simulink model "Spacecraft_Attitude_Dynamics_Control"  (R2020a)
settings: Solver=FixedStepDiscrete  StartTime=0.0  StopTime=300  FixedStep=dt  MaxStep=dt  RelTol=1e-3  EnableMultiTasking=on
InitFcn:
  | % No [0 0 1] %polar orbit
  | 
  | clc
  | close all
  | clear all
  | r0 = [6678;0;0]; %km
  | mu = 398600.4418; % km^3/sec^2
  | v0 = sqrt(mu/norm(r0))*[0;1;0]; % km/s
  | T0 = [0; 0; 0];
  | 
  | I1 = 3;
  | I2 = 4;
  | I3 = 2;
  | I = [I1 0 0; 0 I2 0; 0 0 I3];
  | Iinv  = I ^-1;
  | 
  | k1 = (I1 - I3)/I2;
  | k2 = (I2 - I3)/I1;
  | k3 = (I2 - I1)/I3;
  | n = sqrt(mu/norm(r0)^3);
  | 
  | A11 = zeros(3,3);
  | A12 = (1/2)*eye(3);
  | 
  | F = [-8*k1*n^2 0 0; 0 -6*k2*n^2 0; 0 0 -2*k3*n^2];
  | G = [0 0 (1-k1)*n; 0 0 0; (k3 - 1)*n 0 0];
  | 
  | A = [A11 A12; F G];
  | 
  | B1 = zeros(3,3);
  | B2 =[1/I1 0 0; 0 1/I2 0; 0 0 1/I3];
  | 
  | B = [B1; B2];
  | 
  | Q = [0.32 0 0 0 0 0;
  |        0 0.36 0 0 0 0;
  |        0 0 0.3 0 0 0;
  |        0 0 0 180 0 0;
  |        0 0 0 0 190 0;
  |        0 0 0 0 0 11.5]*10^-4;
  | 
  | 
  | R_LQR = eye(3);
  | 
  | Rinv = R_LQR\eye(3);
  | 
  | S = care(A,B,Q,R_LQR);
  | 
  | K = Rinv*B'*S;
  | 
  | dt = 0.005;
  | dtsim = 0.1;
  | dtdata = 0.01;
  | dtcontrol = 0.2;
  | 
  | Tdist = 0*ones(3,1);
  | Tmin = -0.001; %Nm
  | Tmax = 0.001; %Nm
  | 
  | qTarget = [1;0;0;0];
  | 
  | w0 = [0;0;0]; % Tip: Set w0 to no motion.
  | 
  | H0 = [0;0;0];
  | R = -pi/4;
  | P = pi/4;
  | Y = pi/3;
  | 
  | m = [-0.05; -0.03; -0.05];
  | d = [10; 10 ;10]*(pi/180);
  | 
  | q0 = [cos(R/2)*cos(P/2)*cos(Y/2) - sin(R/2)*sin(P/2)*sin(Y/2);
  |          sin(R/2)*cos(P/2)*cos(Y/2) + cos(R/2)*sin(P/2)*sin(Y/2);
  |          cos(R/2)*sin(P/2)*cos(Y/2) - sin(R/2)*cos(P/2)*sin(Y/2);
  |          cos(R/2)*cos(P/2)*sin(Y/2) + sin(R/2)*sin(P/2)*cos(Y/2)];
  | 
  | 
  | myworld = vrworld('SpacecraftEarth.wrl');
  | open(myworld);
  | set(0,'Units','pixels');
  | scnsize = get(0,'ScreenSize');
  | f1 = vrfigure(myworld,[1 80 scnsize(3)/2 scnsize(4)/2]);
  | set(f1,'Viewpoint','WorldView')
  | f2 = vrfigure(myworld,[scnsize(3)/2 80 scnsize(3)/2 scnsize(4)/2]);
  | set(f2,'Viewpoint','BodyView')
StopFcn:
  | % Roll vs. Time
  | figure
  | 
  | subplot(3,3,1)
  | plot(RPY.time, RPY.signals.values(:,1), '-k');
  | hold on
  | plot([0 RPY.time(end)], 5 *pi/180 * [1,1],'-r');
  | plot([0 RPY.time(end)], -5 *pi/180 * [1,1],'-r');
  | xlabel('Time, sec')
  | ylabel('Roll, rad')
  | xlim([0 RPY.time(end)])
  | hold off
  | 
  | subplot(3,3,2)
  | plot(RPY.time, RPY.signals.values(:,2), '-k');
  | hold on
  | plot([0 RPY.time(end)], 5 *pi/180 * [1,1],'-r');
  | plot([0 RPY.time(end)], -5 *pi/180 * [1,1],'-r');
  | xlabel('Time, sec')
  | ylabel('Pitch, rad')
  | xlim([0 RPY.time(end)])
  | hold off
  | 
  | subplot(3,3,3)
  | plot(RPY.time, RPY.signals.values(:,3), '-k');
  | hold on
  | plot([0 RPY.time(end)], 5 *pi/180 * [1,1],'-r');
  | plot([0 RPY.time(end)], -5 *pi/180 * [1,1],'-r');
  | xlabel('Time, sec')
  | ylabel('Yaw, rad')
  | xlim([0 RPY.time(end)])
  | hold off
  | 
  | % Roll Torque vs. Time
  | subplot(3,3,4)
  | hold on;
  | plot(Torque.time, Torque.signals.values(:,1), '-k');
  | xlabel('Time (seconds)');
  | ylabel('Roll Torque (Newton-Meters)');
  | xlim([0 Torque.time(end)]);
  | 
  | % Pitch Torque vs. Time
  | subplot(3,3,5)
  | hold on;
  | plot(Torque.time, Torque.signals.values(:,2), '-k');
  | xlabel('Time (seconds)');
  | ylabel('Pitch Torque (Newton-Meters)');
  | xlim([0 Torque.time(end)]);
  | 
  | % Yaw Torque vs. Time
  | subplot(3,3,6)
  | hold on;
  | plot(Torque.time, Torque.signals.values(:,3), '-k');
  | xlabel('Time (seconds)');
  | ylabel('Yaw Torque (Newton-Meters)');
  | xlim([0 Torque.time(end)]);
  | 
  | subplot(3,3,7)
  | hold on;
  | plot(thetaError.signals.values(:,1),thetaDot.signals.values(:,1),'-k');
  | axis manual;
  | pause(0.1);
  | plot([-2 2], [m(1)*-2+m(1)*d(1)/2, m(1)*2+m(1)*d(1)/2],'-r');
  | plot([-2 2], [m(1)*-2-m(1)*d(1)/2, m(1)*2-m(1)*d(1)/2],'-r');
  | 
  | 
  | subplot(3,3,8)
  | hold on;
  | plot(thetaError.signals.values(:,2),thetaDot.signals.values(:,2),'-k');
  | axis manual;
  | pause(0.1);
  | plot([-2 2], [m(2)*-2+m(2)*d(2)/2, m(2)*2+m(2)*d(2)/2],'-r');
  | plot([-2 2], [m(2)*-2-m(2)*d(2)/2, m(2)*2-m(2)*d(2)/2],'-r');
  | 
  | 
  | subplot(3,3,9)
  | hold on;
  | plot(thetaError.signals.values(:,3),thetaDot.signals.values(:,3),'-k');
  | axis manual;
  | pause(0.1);
  | plot([-2 2], [m(3)*-2+m(3)*d(3)/2, m(3)*2+m(3)*d(3)/2],'-r');
  | plot([-2 2], [m(3)*-2-m(3)*d(3)/2, m(3)*2-m(3)*d(3)/2],'-r');
  | hold off
  | 
  | 
  | titletext = ['Cost Function J = ' num2str(J.signals.values(end))];
  | sgtitle(titletext)
  | fprintf('%d %d %d \n',abs(RPY.signals.values(end,:)*180/pi)<0.1)
  | fprintf('%d %d %d \n',abs(thetaDot.signals.values(end,1:3))<1e-4)
  | display(RPY.signals.values(end,:)*180/pi)
  | display(thetaDot.signals.values(end,1:3))
undefined symbols (not defined in the file): DiscIntNeverNeededParam
libraries: sharedutil x5, vrlib x1, simulink x1
settings Model: Creator=HANE  LastModifiedBy=Edward Han
settings DataIOCC: ReturnWorkspaceOutputs=off
settings DebuggingCC: SFExecutionAtInitializationDiag=none  ArithmeticOperatorsInVariantConditions=warning
settings SFSimCC: SimUseLocalCustomCode=off  CustomCodeUndefinedFunction=UseInterfaceOnly
settings RTWCC: RTWUseLocalCustomCode=off
settings CodeAppCC: StateflowObjectComments=on

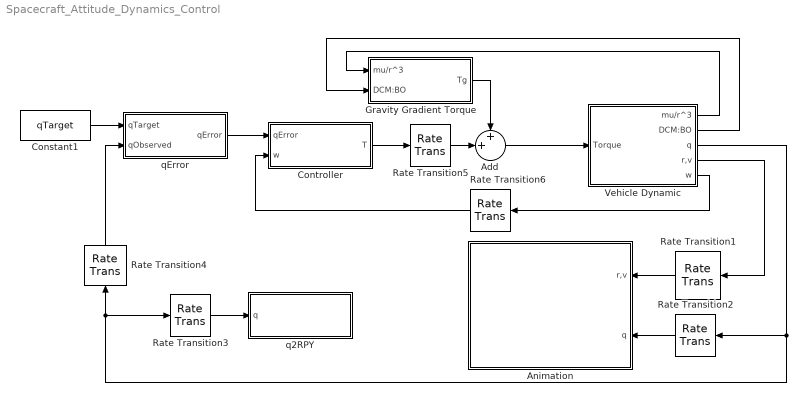
== system Spacecraft_Attitude_Dynamics_Control ==
  Add : Sum  Inputs=++|
  Animation : Subsystem
  Constant1 : Constant  Value=qTarget
  Controller : Subsystem
  Gravity Gradient Torque : Subsystem
  Rate Transition1 : RateTransition  InitialCondition=[r0;v0]  OutPortSampleTime=dtsim
  Rate Transition2 : RateTransition  InitialCondition=q0  OutPortSampleTime=dtsim
  Rate Transition3 : RateTransition  InitialCondition=q0  OutPortSampleTime=dtdata
  Rate Transition4 : RateTransition  InitialCondition=q0  OutPortSampleTime=dtcontrol
  Rate Transition5 : RateTransition  InitialCondition=T0  OutPortSampleTime=dt
  Rate Transition6 : RateTransition  InitialCondition=w0  OutPortSampleTime=dtcontrol
  Vehicle Dynamic : Subsystem
  q2RPY : Subsystem
  qError : Subsystem
  wires:
  Add/1 -> Vehicle Dynamic/1(Torque)
  Vehicle Dynamic/4(r,v) -> Rate Transition1/1
  Vehicle Dynamic/3(q) -> Rate Transition3/1, Rate Transition4/1, Rate Transition2/1
  Rate Transition2/1 -> Animation/2(q)
  Rate Transition1/1 -> Animation/1(r,v)
  Rate Transition3/1 -> q2RPY/1(q)
  Rate Transition5/1 -> Add/2
  Controller/1(T) -> Rate Transition5/1
  Constant1/1 -> qError/1(qTarget)
  qError/1(qError) -> Controller/1(qError)
  Rate Transition4/1 -> qError/2(qObserved)
  Vehicle Dynamic/5(w) -> Rate Transition6/1
  Vehicle Dynamic/1(mu/r^3) -> Gravity Gradient Torque/1(mu/r^3)
  Vehicle Dynamic/2(DCM:BO) -> Gravity Gradient Torque/2(DCM:BO)
  Gravity Gradient Torque/1(Tg) -> Add/1
  Rate Transition6/1 -> Controller/2("w ")

== system Spacecraft_Attitude_Dynamics_Control/Animation ==
  r,v : Inport
  q : Inport  Port=2
  Demux : Demux  Outputs=[3,3]
  Earth Rotation : Subsystem
  VR Sink : vrlib/VR Sink  InstantiateOnLoad=on  SampleTime=dtsim  ViewEnable=on  RemoteChange=off  RemoteView=off  FieldsWritten=Earth.rotation.4.1.1.double#BodyView.orientation.4.1.1.double#BodyView.position.3.1.1.double#Spacecraft.rotation.4.1.1.double#Spacecraft.translation.3.1.1.double  WorldFileName=SpacecraftEarth.wrl  AutoView=off  VideoDimensions=[]  AllowVariableSize=off
  q2eulerparameters : Subsystem
  qBody wrt Inertial : Subsystem
  qOrbit wrt Inertial : Subsystem
  qOrbit wrt Inertial1 : Subsystem
  "r, translation" : Subsystem
  wires:
  Demux/1 -> qOrbit wrt Inertial/1(r), "r, translation"/1(r), qOrbit wrt Inertial1/1(r)
  Demux/2 -> qOrbit wrt Inertial/2(v)
  q/1 -> qBody wrt Inertial/2(qBO)
  qOrbit wrt Inertial/2("qOI ") -> qBody wrt Inertial/1(qOI)
  qBody wrt Inertial/1(qBI) -> q2eulerparameters/1(q)
  r,v/1 -> Demux/1
  "r, translation"/1(translation) -> VR Sink/5
  qOrbit wrt Inertial/1(DCM) -> qOrbit wrt Inertial1/2(DCM)
  Earth Rotation/1(Earth Rotation) -> VR Sink/1
  qOrbit wrt Inertial1/1(Nadir View Rotation) -> VR Sink/2
  qOrbit wrt Inertial1/2(Nadir View Position) -> VR Sink/3
  q2eulerparameters/1(e,phi) -> VR Sink/4

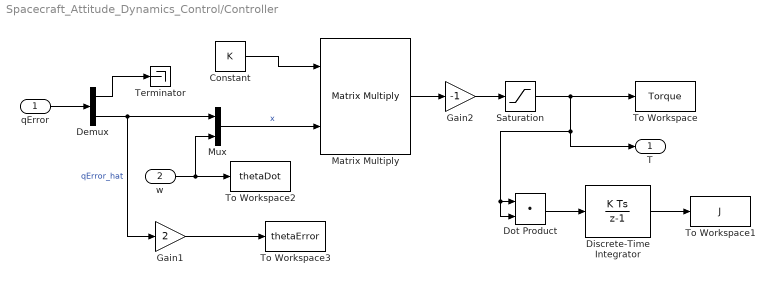
== system Spacecraft_Attitude_Dynamics_Control/Controller ==
  qError : Inport  SampleTime=dtcontrol
  "w " : Inport  Port=2
  Constant : Constant  Value=K
  Demux : Demux  Outputs=[1,3]
  Discrete-Time Integrator : DiscreteIntegrator  SampleTime=dtcontrol  ICPrevOutput=DiscIntNeverNeededParam  ICPrevScaledInput=DiscIntNeverNeededParam
  Dot Product : DotProduct  InputSameDT=on  OutDataTypeStr=Inherit: Inherit via internal rule
  Gain1 : Gain  Gain=2
  Gain2 : Gain  Gain=-1
  Matrix Multiply : Product  Multiplication=Matrix(*)
  Mux : Mux  Inputs=2
  Saturation : Saturate  UpperLimit=Tmax  LowerLimit=-Tmax
  Terminator : Terminator
  To Workspace : ToWorkspace  VariableName=Torque  SaveFormat=Structure With Time  SampleTime=-1
  To Workspace1 : ToWorkspace  VariableName=J  SaveFormat=Structure With Time  SampleTime=-1
  To Workspace2 : ToWorkspace  VariableName=thetaDot  SaveFormat=Structure With Time  SampleTime=-1
  To Workspace3 : ToWorkspace  VariableName=thetaError  SaveFormat=Structure With Time  SampleTime=-1
  T : Outport  VectorParamsAs1DForOutWhenUnconnected=off
  wires:
  qError/1 -> Demux/1
  "w "/1 -> To Workspace2/1, Mux/2
  Demux/2 -> Gain1/1, Mux/1  "qError_hat"
  Demux/1 -> Terminator/1
  Mux/1 -> Matrix Multiply/2  "x"
  Matrix Multiply/1 -> Gain2/1
  Gain2/1 -> Saturation/1
  Dot Product/1 -> Discrete-Time Integrator/1
  Discrete-Time Integrator/1 -> To Workspace1/1
  Constant/1 -> Matrix Multiply/1
  Gain1/1 -> To Workspace3/1
  Saturation/1 -> To Workspace/1, Dot Product/2, Dot Product/1, T/1

== system Spacecraft_Attitude_Dynamics_Control/Gravity Gradient Torque ==
  mu/r^3 : Inport
  DCM:BO : Inport  Port=2
  3x3 Cross Product : sharedutil/3x3 Cross Product  aMode=aMode
      settings: SourceProductBaseCode=AE,PW,MT,VE,VP
  Constant : Constant  Value=[0;0;-1]
  Gain : Gain  Gain=3
  "I " : Constant  Value=I
  Matrix Multiply : Product  Multiplication=Matrix(*)
  Multiply : Product
  Multiply1 : Product  Multiplication=Matrix(*)
  Tg : Outport  VectorParamsAs1DForOutWhenUnconnected=off
  wires:
  mu/r^3/1 -> Gain/1
  DCM:BO/1 -> Matrix Multiply/1
  Constant/1 -> Matrix Multiply/2
  Matrix Multiply/1 -> Multiply1/2, Multiply/2  "rhat"
  Gain/1 -> Multiply/1
  Multiply/1 -> 3x3 Cross Product/1
  3x3 Cross Product/1 -> Tg/1
  "I "/1 -> Multiply1/1
  Multiply1/1 -> 3x3 Cross Product/2

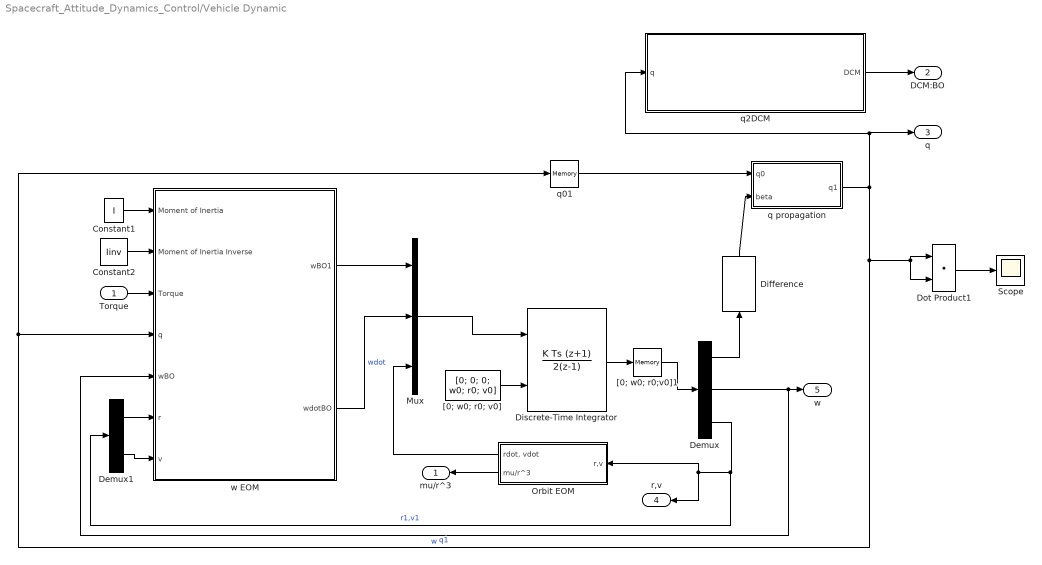
== system Spacecraft_Attitude_Dynamics_Control/Vehicle Dynamic ==
  Torque : Inport
  Constant1 : Constant  Value=I
  Constant2 : Constant  Value=Iinv
  Demux : Demux  Outputs=[3,3,6]
  Demux1 : Demux  Outputs=2
  Difference : simulink/Discrete/Difference  ICPrevInput=0.0  OutMin=[]  OutMax=[]  OutDataType=fixdt(1, 16)  OutScaling=2^-10  DoSatur=off
  Discrete-Time Integrator : DiscreteIntegrator  IntegratorMethod=Integration: Trapezoidal  InitialConditionSource=external  SampleTime=dt  ICPrevOutput=DiscIntNeverNeededParam  ICPrevScaledInput=DiscIntNeverNeededParam
  Dot Product1 : DotProduct  InputSameDT=on  OutDataTypeStr=Inherit: Inherit via internal rule
  Mux : Mux  Inputs=3
  Orbit EOM : Subsystem
  Scope : Scope
  "[0; w0; r0; v0]" : Constant  Value=[0; 0; 0; w0; r0; v0]
  "[0; w0; r0;v0]1" : Memory  InitialCondition=[0; 0; 0; w0; r0; v0]  InheritSampleTime=on
  q propagation : Subsystem
  q01 : Memory  InitialCondition=q0  InheritSampleTime=on
  q2DCM : Subsystem
  w EOM : Subsystem
  mu/r^3 : Outport  VectorParamsAs1DForOutWhenUnconnected=off
  DCM:BO : Outport  Port=2  VectorParamsAs1DForOutWhenUnconnected=off
  q : Outport  Port=3  VectorParamsAs1DForOutWhenUnconnected=off
  r,v : Outport  Port=4  VectorParamsAs1DForOutWhenUnconnected=off
  w : Outport  Port=5  VectorParamsAs1DForOutWhenUnconnected=off
  wires:
  Mux/1 -> Discrete-Time Integrator/1
  Demux/3 -> Demux1/1, Orbit EOM/1(r,v), r,v/1  "r1,v1"
  Constant1/1 -> w EOM/1(Moment of Inertia)
  "[0; w0; r0;v0]1"/1 -> Demux/1
  "[0; w0; r0; v0]"/1 -> Discrete-Time Integrator/2
  Orbit EOM/1("rdot, vdot ") -> Mux/3
  Torque/1 -> w EOM/3(Torque)
  q propagation/1(q1) -> Dot Product1/1, Dot Product1/2, q01/1, w EOM/4(q), q/1, q2DCM/1(q)  "q1"
  Difference/1 -> q propagation/2(beta)
  q01/1 -> q propagation/1(q0)
  Constant2/1 -> w EOM/2(Moment of Inertia Inverse)
  Dot Product1/1 -> Scope/1
  Discrete-Time Integrator/1 -> "[0; w0; r0;v0]1"/1
  w EOM/2(wdotBO) -> Mux/2  "wdot"
  Demux1/2 -> w EOM/7("v ")
  Demux1/1 -> w EOM/6(r)
  Demux/2 -> w/1, w EOM/5("wBO ")  "w"
  Demux/1 -> Difference/1
  w EOM/1(wBO1) -> Mux/1
  q2DCM/1(DCM) -> DCM:BO/1
  Orbit EOM/2(mu/r^3) -> mu/r^3/1

== system Spacecraft_Attitude_Dynamics_Control/q2RPY ==
  q : Inport
  DCM(1,1) : Fcn  Expr=(u(1)^2+u(2)^2-u(3)^2-u(4)^2)
  DCM(2,1) : Fcn  Expr=2*(u(2)*u(3)-u(4)*u(1))
  DCM(3,1) : Fcn  Expr=2*(u(2)*u(4)+u(1)*u(3))
  DCM(3,2) : Fcn  Expr=2*(u(3)*u(4)-u(1)*u(2))
  DCM(3,3) : Fcn  Expr=(u(1)^2-u(2)^2-u(3)^2+u(4)^2)
  Gain : Gain  Gain=-1
  Gain1 : Gain  Gain=-1
  Mux : Mux  Inputs=3
  To Workspace : ToWorkspace  VariableName=RPY  SaveFormat=Structure With Time  SampleTime=-1
  Trigonometric Function : Trigonometry  Operator=asin
  Trigonometric Function1 : Trigonometry  Operator=atan2
  Trigonometric Function2 : Trigonometry  Operator=atan2
  wires:
  q/1 -> DCM(1,1)/1, DCM(2,1)/1, DCM(3,3)/1, DCM(3,2)/1, DCM(3,1)/1
  DCM(3,1)/1 -> Trigonometric Function/1
  DCM(3,3)/1 -> Trigonometric Function1/2
  Trigonometric Function1/1 -> Mux/1  "R"
  Trigonometric Function/1 -> Mux/2  "P"
  DCM(1,1)/1 -> Trigonometric Function2/2
  Trigonometric Function2/1 -> Mux/3  "Y"
  Mux/1 -> To Workspace/1
  Gain/1 -> Trigonometric Function2/1
  DCM(2,1)/1 -> Gain/1
  DCM(3,2)/1 -> Gain1/1
  Gain1/1 -> Trigonometric Function1/1

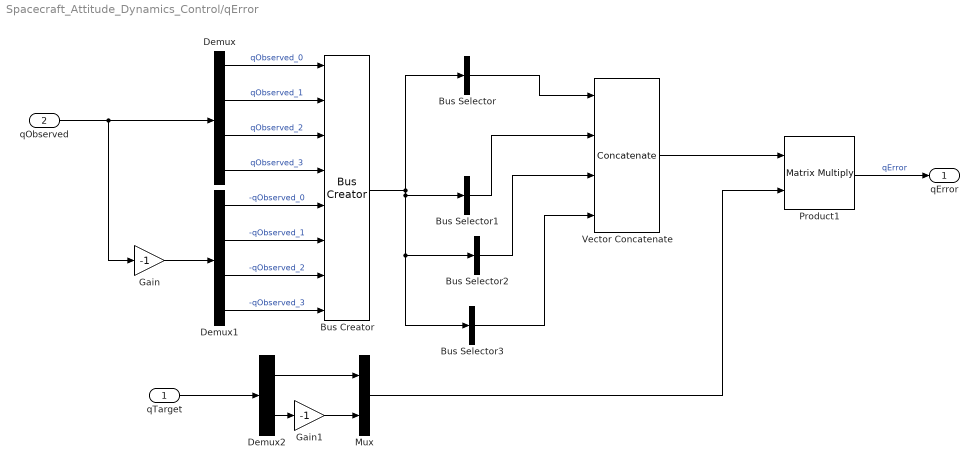
== system Spacecraft_Attitude_Dynamics_Control/qError ==
  qTarget : Inport
  qObserved : Inport  Port=2
  Bus Creator : BusCreator  Inputs=8
  Bus Selector : BusSelector  OutputSignals=qObserved_0,qObserved_1,qObserved_2,qObserved_3  OutputAsBus=on
  Bus Selector1 : BusSelector  OutputSignals=-qObserved_1,qObserved_0,-qObserved_3,qObserved_2  OutputAsBus=on
  Bus Selector2 : BusSelector  OutputSignals=-qObserved_2,qObserved_3,qObserved_0,-qObserved_1  OutputAsBus=on
  Bus Selector3 : BusSelector  OutputSignals=-qObserved_3,-qObserved_2,qObserved_1,qObserved_0  OutputAsBus=on
  Demux : Demux
  Demux1 : Demux
  Demux2 : Demux  Outputs=[1,3]
  Gain : Gain  Gain=-1
  Gain1 : Gain  Gain=-1
  Mux : Mux  Inputs=2
  Product1 : Product  Multiplication=Matrix(*)
  Vector Concatenate : Concatenate  NumInputs=4  Mode=Multidimensional array  ConcatenateDimension=2
  qError : Outport  VectorParamsAs1DForOutWhenUnconnected=off
  wires:
  qObserved/1 -> Gain/1, Demux/1
  Bus Selector3/1 -> Vector Concatenate/4
  Bus Selector2/1 -> Vector Concatenate/3
  Bus Creator/1 -> Bus Selector/1, Bus Selector2/1, Bus Selector3/1, Bus Selector1/1
  Demux1/2 -> Bus Creator/6  "-qObserved_1"
  Mux/1 -> Product1/2
  Product1/1 -> qError/1  "qError"
  Vector Concatenate/1 -> Product1/1
  Demux/2 -> Bus Creator/2  "qObserved_1"
  Bus Selector1/1 -> Vector Concatenate/2
  Demux1/1 -> Bus Creator/5  "-qObserved_0"
  Demux1/4 -> Bus Creator/8  "-qObserved_3"
  Demux/4 -> Bus Creator/4  "qObserved_3"
  Demux/3 -> Bus Creator/3  "qObserved_2"
  Gain/1 -> Demux1/1
  Bus Selector/1 -> Vector Concatenate/1
  Demux/1 -> Bus Creator/1  "qObserved_0"
  Demux1/3 -> Bus Creator/7  "-qObserved_2"
  qTarget/1 -> Demux2/1
  Demux2/2 -> Gain1/1
  Demux2/1 -> Mux/1
  Gain1/1 -> Mux/2

== system Spacecraft_Attitude_Dynamics_Control/Animation/Earth Rotation ==
  Cos : Trigonometry  Operator=cos
  Digital Clock : DigitalClock  SampleTime=dtsim
  Gain : Gain  Gain=1/2
  Gain1 : Gain  Gain=1/sqrt(2)
  Mux : Mux
  Product : Product
  Sin : Trigonometry
  q2eulerparameters : Subsystem
  w Earth : Constant  Value=2*pi/(24*3600)
  Earth Rotation : Outport  VectorParamsAs1DForOutWhenUnconnected=off
  wires:
  Gain1/1 -> q2eulerparameters/1(q)
  Cos/1 -> Mux/2, Mux/1
  Sin/1 -> Mux/4, Mux/3
  Mux/1 -> Gain1/1
  q2eulerparameters/1(e,phi) -> Earth Rotation/1
  Gain/1 -> Sin/1, Cos/1
  Product/1 -> Gain/1
  w Earth/1 -> Product/2
  Digital Clock/1 -> Product/1

== system Spacecraft_Attitude_Dynamics_Control/Animation/q2eulerparameters ==
  q : Inport
  Demux : Demux  Outputs=[1,3]
  Divide : Product  Inputs=/*
  Gain : Gain  Gain=2
  Mux : Mux  Inputs=2
  Trigonometric Function : Trigonometry  Operator=acos
  Trigonometric Function1 : Trigonometry
  e,phi : Outport  VectorParamsAs1DForOutWhenUnconnected=off
  wires:
  Demux/2 -> Divide/2  "qhat"
  Trigonometric Function1/1 -> Divide/1
  Divide/1 -> Mux/1  "e"
  Trigonometric Function/1 -> Trigonometric Function1/1, Gain/1  "phi/2"
  Demux/1 -> Trigonometric Function/1  "q0"
  Gain/1 -> Mux/2  "phi"
  Mux/1 -> e,phi/1
  q/1 -> Demux/1

== system Spacecraft_Attitude_Dynamics_Control/Animation/qBody wrt Inertial ==
  qOI : Inport
  qBO : Inport  Port=2
  Bus Creator : BusCreator  Inputs=8
  Bus Selector : BusSelector  OutputSignals=qBO_0,qBO_1,qBO_2,qBO_3  OutputAsBus=on
  Bus Selector1 : BusSelector  OutputSignals=-qBO_1,qBO_0,-qBO_3,qBO_2  OutputAsBus=on
  Bus Selector2 : BusSelector  OutputSignals=-qBO_2,qBO_3,qBO_0,-qBO_1  OutputAsBus=on
  Bus Selector3 : BusSelector  OutputSignals=-qBO_3,-qBO_2,qBO_1,qBO_0  OutputAsBus=on
  Demux : Demux
  Demux1 : Demux
  Gain : Gain  Gain=-1
  Product1 : Product  Multiplication=Matrix(*)
  Vector Concatenate : Concatenate  NumInputs=4  Mode=Multidimensional array  ConcatenateDimension=2
  qBI : Outport  VectorParamsAs1DForOutWhenUnconnected=off
  wires:
  qBO/1 -> Demux/1, Gain/1
  Demux/1 -> Bus Creator/1  "qBO_0"
  Gain/1 -> Demux1/1
  Demux/2 -> Bus Creator/2  "qBO_1"
  Demux/3 -> Bus Creator/3  "qBO_2"
  Demux/4 -> Bus Creator/4  "qBO_3"
  Demux1/1 -> Bus Creator/5  "-qBO_0"
  Demux1/2 -> Bus Creator/6  "-qBO_1"
  Demux1/3 -> Bus Creator/7  "-qBO_2"
  Demux1/4 -> Bus Creator/8  "-qBO_3"
  Bus Creator/1 -> Bus Selector3/1, Bus Selector2/1, Bus Selector1/1, Bus Selector/1
  Bus Selector3/1 -> Vector Concatenate/4
  Bus Selector2/1 -> Vector Concatenate/3
  Bus Selector1/1 -> Vector Concatenate/2
  Bus Selector/1 -> Vector Concatenate/1
  Vector Concatenate/1 -> Product1/1
  qOI/1 -> Product1/2
  Product1/1 -> qBI/1  "qBI"

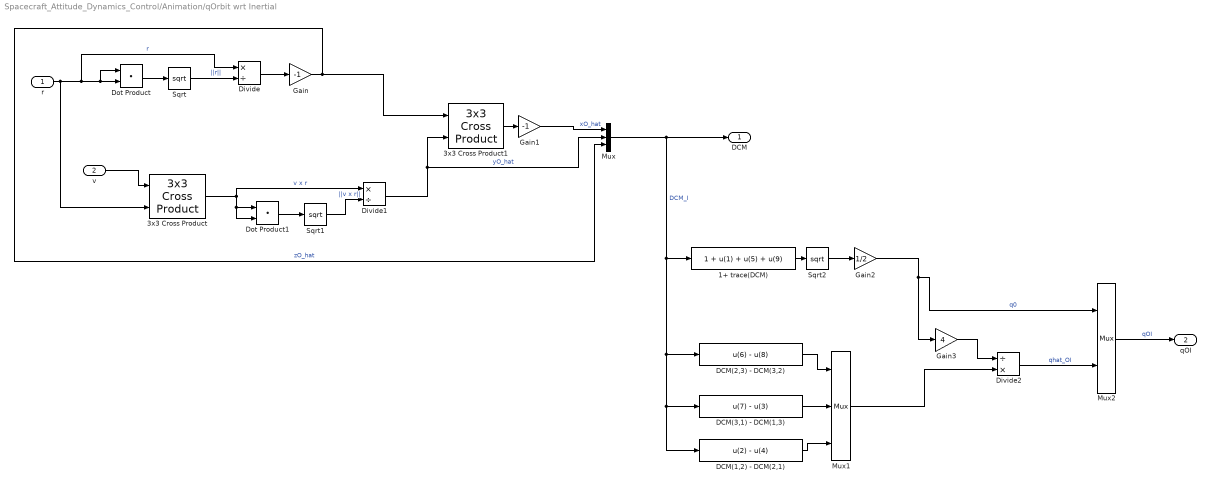
== system Spacecraft_Attitude_Dynamics_Control/Animation/qOrbit wrt Inertial ==
  r : Inport
  v : Inport  Port=2
  "1+ trace(DCM) " : Fcn  Expr=1 + u(1) + u(5) + u(9)
  3x3 Cross Product : sharedutil/3x3 Cross Product  aMode=aMode
      settings: SourceProductBaseCode=AE,PW,MT,VE,VP
  3x3 Cross Product1 : sharedutil/3x3 Cross Product  aMode=aMode
      settings: SourceProductBaseCode=AE,PW,MT,VE,VP
  DCM(1,2) - DCM(2,1) : Fcn  Expr=u(2) - u(4)
  DCM(2,3) - DCM(3,2) : Fcn  Expr=u(6) - u(8)
  DCM(3,1) - DCM(1,3) : Fcn  Expr=u(7) - u(3)
  Divide : Product  Inputs=*/
  Divide1 : Product  Inputs=*/
  Divide2 : Product  Inputs=/*
  Dot Product : DotProduct  InputSameDT=on  OutDataTypeStr=Inherit: Inherit via internal rule
  Dot Product1 : DotProduct  InputSameDT=on  OutDataTypeStr=Inherit: Inherit via internal rule
  Gain : Gain  Gain=-1
  Gain1 : Gain  Gain=-1
  Gain2 : Gain  Gain=1/2
  Gain3 : Gain  Gain=4
  Mux : Mux  Inputs=3
  Mux1 : Mux  Inputs=3
  Mux2 : Mux  Inputs=2
  Sqrt : Sqrt  SaturateOnIntegerOverflow=on
  Sqrt1 : Sqrt  SaturateOnIntegerOverflow=on
  Sqrt2 : Sqrt  SaturateOnIntegerOverflow=on
  DCM : Outport  VectorParamsAs1DForOutWhenUnconnected=off
  "qOI " : Outport  Port=2  VectorParamsAs1DForOutWhenUnconnected=off
  wires:
  Sqrt/1 -> Divide/2  "||r||"
  r/1 -> 3x3 Cross Product/2, Divide/1, Dot Product/1, Dot Product/2  "r"
  Dot Product/1 -> Sqrt/1
  Divide/1 -> Gain/1
  Gain/1 -> 3x3 Cross Product1/1, Mux/3  "zO_hat"
  v/1 -> 3x3 Cross Product/1
  Dot Product1/1 -> Sqrt1/1
  Sqrt1/1 -> Divide1/2  "||v x r||"
  3x3 Cross Product/1 -> Dot Product1/1, Dot Product1/2, Divide1/1  "v x r"
  Divide1/1 -> 3x3 Cross Product1/2, Mux/2  "yO_hat"
  3x3 Cross Product1/1 -> Gain1/1
  Gain1/1 -> Mux/1  "xO_hat"
  Mux/1 -> DCM(3,1) - DCM(1,3)/1, DCM(1,2) - DCM(2,1)/1, DCM(2,3) - DCM(3,2)/1, "1+ trace(DCM) "/1, DCM/1  "DCM_I"
  "1+ trace(DCM) "/1 -> Sqrt2/1
  Sqrt2/1 -> Gain2/1
  Gain2/1 -> Mux2/1, Gain3/1  "q0"
  DCM(2,3) - DCM(3,2)/1 -> Mux1/1
  DCM(3,1) - DCM(1,3)/1 -> Mux1/2
  DCM(1,2) - DCM(2,1)/1 -> Mux1/3
  Gain3/1 -> Divide2/1
  Mux1/1 -> Divide2/2
  Divide2/1 -> Mux2/2  "qhat_OI"
  Mux2/1 -> "qOI "/1  "qOI"

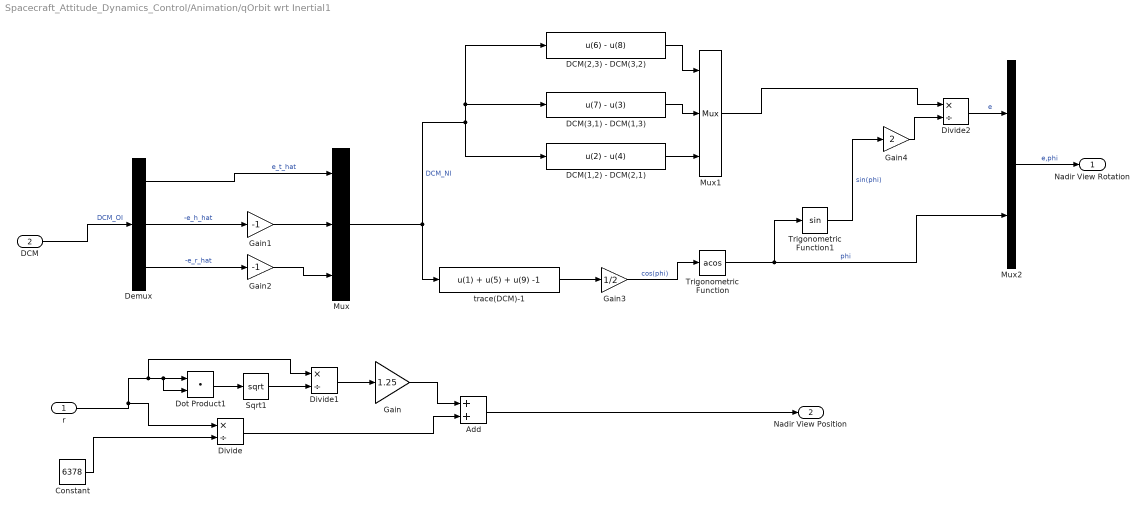
== system Spacecraft_Attitude_Dynamics_Control/Animation/qOrbit wrt Inertial1 ==
  r : Inport
  DCM : Inport  Port=2
  Add : Sum
  Constant : Constant  Value=6378
  DCM(1,2) - DCM(2,1) : Fcn  Expr=u(2) - u(4)
  DCM(2,3) - DCM(3,2) : Fcn  Expr=u(6) - u(8)
  DCM(3,1) - DCM(1,3) : Fcn  Expr=u(7) - u(3)
  Demux : Demux  Outputs=[3,3,3]
  Divide : Product  Inputs=*/
  Divide1 : Product  Inputs=*/
  Divide2 : Product  Inputs=*/
  Dot Product1 : DotProduct  InputSameDT=on  OutDataTypeStr=Inherit: Inherit via internal rule
  Gain : Gain  Gain=1.25
  Gain1 : Gain  Gain=-1
  Gain2 : Gain  Gain=-1
  Gain3 : Gain  Gain=1/2
  Gain4 : Gain  Gain=2
  Mux : Mux  Inputs=3
  Mux1 : Mux  Inputs=3
  Mux2 : Mux  Inputs=2
  Sqrt1 : Sqrt  SaturateOnIntegerOverflow=on
  Trigonometric Function : Trigonometry  Operator=acos
  Trigonometric Function1 : Trigonometry
  "trace(DCM)-1 " : Fcn  Expr=u(1) + u(5) + u(9) -1
  Nadir View Rotation : Outport  VectorParamsAs1DForOutWhenUnconnected=off
  Nadir View Position : Outport  Port=2  VectorParamsAs1DForOutWhenUnconnected=off
  wires:
  Constant/1 -> Divide/2
  Add/1 -> Nadir View Position/1
  r/1 -> Divide1/1, Dot Product1/2, Dot Product1/1, Divide/1
  Divide/1 -> Add/2
  Sqrt1/1 -> Divide1/2
  Dot Product1/1 -> Sqrt1/1
  Divide1/1 -> Gain/1
  Gain/1 -> Add/1
  DCM/1 -> Demux/1  "DCM_OI"
  Demux/1 -> Mux/1  "e_t_hat"
  Demux/2 -> Gain1/1  "-e_h_hat"
  Demux/3 -> Gain2/1  "-e_r_hat"
  Gain1/1 -> Mux/2
  Gain2/1 -> Mux/3
  Mux/1 -> DCM(3,1) - DCM(1,3)/1, DCM(2,3) - DCM(3,2)/1, DCM(1,2) - DCM(2,1)/1, "trace(DCM)-1 "/1  "DCM_NI"
  DCM(3,1) - DCM(1,3)/1 -> Mux1/2
  "trace(DCM)-1 "/1 -> Gain3/1
  DCM(1,2) - DCM(2,1)/1 -> Mux1/3
  Divide2/1 -> Mux2/1  "e"
  DCM(2,3) - DCM(3,2)/1 -> Mux1/1
  Gain3/1 -> Trigonometric Function/1  "cos(phi)"
  Trigonometric Function/1 -> Mux2/2, Trigonometric Function1/1  "phi"
  Trigonometric Function1/1 -> Gain4/1  "sin(phi)"
  Gain4/1 -> Divide2/2
  Mux1/1 -> Divide2/1
  Mux2/1 -> Nadir View Rotation/1  "e,phi"

== system Spacecraft_Attitude_Dynamics_Control/Animation/r, translation ==
  r : Inport
  Constant : Constant  Value=6378
  Divide : Product  Inputs=*/
  translation : Outport  VectorParamsAs1DForOutWhenUnconnected=off
  wires:
  r/1 -> Divide/1
  Divide/1 -> translation/1
  Constant/1 -> Divide/2

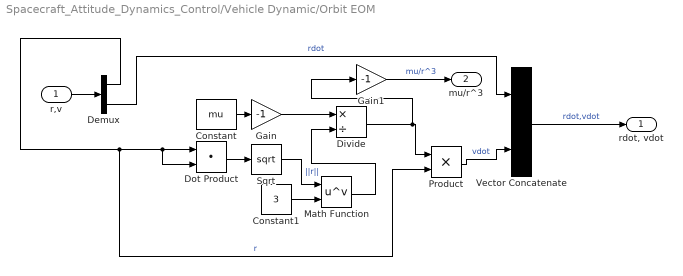
== system Spacecraft_Attitude_Dynamics_Control/Vehicle Dynamic/Orbit EOM ==
  r,v : Inport
  Constant : Constant  Value=mu
  Constant1 : Constant  Value=3
  Demux : Demux  Outputs=[3,3]
  Divide : Product  Inputs=*/
  Dot Product : DotProduct  InputSameDT=on  OutDataTypeStr=Inherit: Inherit via internal rule
  Gain : Gain  Gain=-1
  Gain1 : Gain  Gain=-1
  Math Function : Math  Operator=pow  SignedPower=on  SaturateOnIntegerOverflow=on
  Product : Product
  Sqrt : Sqrt  SaturateOnIntegerOverflow=on
  Vector Concatenate : Concatenate
  "rdot, vdot " : Outport  VectorParamsAs1DForOutWhenUnconnected=off
  mu/r^3 : Outport  Port=2  VectorParamsAs1DForOutWhenUnconnected=off
  wires:
  Dot Product/1 -> Sqrt/1
  Sqrt/1 -> Math Function/1  "||r||"
  Constant1/1 -> Math Function/2
  Math Function/1 -> Divide/2
  Constant/1 -> Gain/1
  Gain/1 -> Divide/1
  Divide/1 -> Gain1/1, Product/1
  Product/1 -> Vector Concatenate/2  "vdot"
  Vector Concatenate/1 -> "rdot, vdot "/1  "rdot,vdot"
  r,v/1 -> Demux/1
  Demux/1 -> Product/2, Dot Product/2, Dot Product/1  "r"
  Demux/2 -> Vector Concatenate/1  "rdot"
  Gain1/1 -> mu/r^3/1  "mu/r^3"

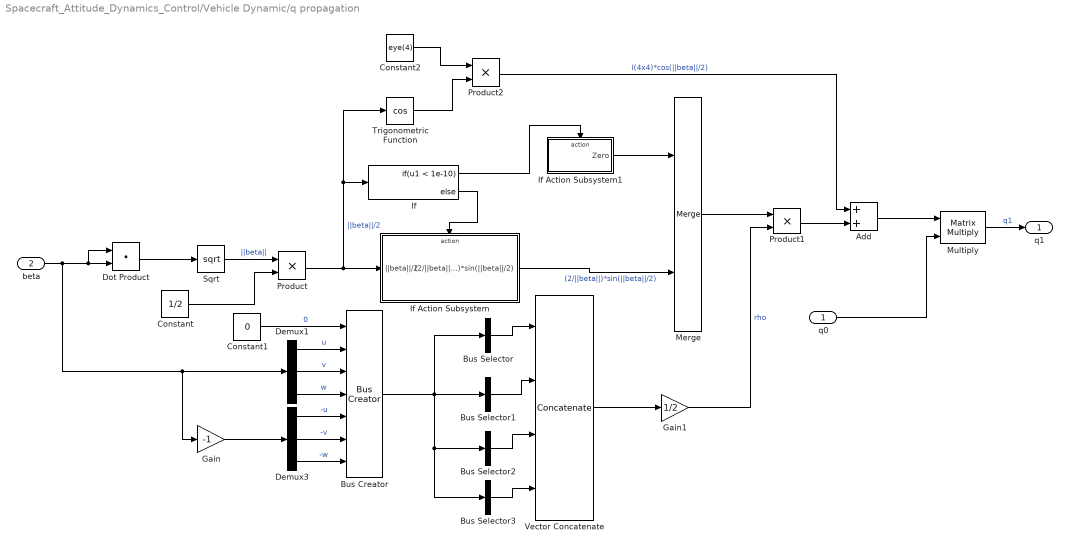
== system Spacecraft_Attitude_Dynamics_Control/Vehicle Dynamic/q propagation ==
  q0 : Inport
  beta : Inport  Port=2
  Add : Sum
  Bus Creator : BusCreator  Inputs=7
  Bus Selector : BusSelector  OutputSignals=0,u,v,w  OutputAsBus=on
  Bus Selector1 : BusSelector  OutputSignals=-u,0,-w,v  OutputAsBus=on
  Bus Selector2 : BusSelector  OutputSignals=-v,w,0,-u  OutputAsBus=on
  Bus Selector3 : BusSelector  OutputSignals=-w,-v,u,0  OutputAsBus=on
  Constant : Constant  Value=1/2
  Constant1 : Constant  Value=0
  Constant2 : Constant  Value=eye(4)
  Demux1 : Demux  Outputs=3
      settings: DisplayOption=none
  Demux3 : Demux  Outputs=3
      settings: DisplayOption=none
  Dot Product : DotProduct  InputSameDT=on  OutDataTypeStr=Inherit: Inherit via internal rule
  Gain : Gain  Gain=-1
  Gain1 : Gain  Gain=1/2
  If : If  IfExpression=u1 < 1e-10
  If Action Subsystem : Subsystem  TreatAsAtomicUnit=on
  If Action Subsystem1 : Subsystem  TreatAsAtomicUnit=on
  Merge : Merge
  Multiply : Product  Multiplication=Matrix(*)
  Product : Product
  Product1 : Product
  Product2 : Product
  Sqrt : Sqrt  SaturateOnIntegerOverflow=on
  Trigonometric Function : Trigonometry  Operator=cos
  Vector Concatenate : Concatenate  NumInputs=4  Mode=Multidimensional array  ConcatenateDimension=2
  q1 : Outport  VectorParamsAs1DForOutWhenUnconnected=off
  wires:
  If/1 -> If Action Subsystem1/Action
  If/2 -> If Action Subsystem/Action
  Merge/1 -> Product1/1
  If Action Subsystem1/1(Zero) -> Merge/1
  Product/1 -> Trigonometric Function/1, If/1, If Action Subsystem/1(||beta||/2)  "||beta||/2"
  If Action Subsystem/1((2/||beta||)*sin(||beta||/2)) -> Merge/2  "(2/||beta||)*sin(||beta||/2)"
  Sqrt/1 -> Product/1  "||beta||"
  beta/1 -> Gain/1, Demux1/1, Dot Product/1, Dot Product/2
  Dot Product/1 -> Sqrt/1
  Constant/1 -> Product/2
  Gain/1 -> Demux3/1
  Demux1/2 -> Bus Creator/3  "v"
  Demux1/1 -> Bus Creator/2  "u"
  Demux1/3 -> Bus Creator/4  "w"
  Demux3/1 -> Bus Creator/5  "-u"
  Demux3/2 -> Bus Creator/6  "-v"
  Demux3/3 -> Bus Creator/7  "-w"
  Constant1/1 -> Bus Creator/1  "0"
  Bus Creator/1 -> Bus Selector3/1, Bus Selector2/1, Bus Selector1/1, Bus Selector/1
  Bus Selector/1 -> Vector Concatenate/1
  Bus Selector1/1 -> Vector Concatenate/2
  Bus Selector2/1 -> Vector Concatenate/3
  Bus Selector3/1 -> Vector Concatenate/4
  Vector Concatenate/1 -> Gain1/1
  Gain1/1 -> Product1/2  "rho"
  Constant2/1 -> Product2/1
  Trigonometric Function/1 -> Product2/2
  Product2/1 -> Add/1  "I(4x4)*cos(||beta||/2)"
  Product1/1 -> Add/2
  Add/1 -> Multiply/1
  q0/1 -> Multiply/2
  Multiply/1 -> q1/1  "q1"

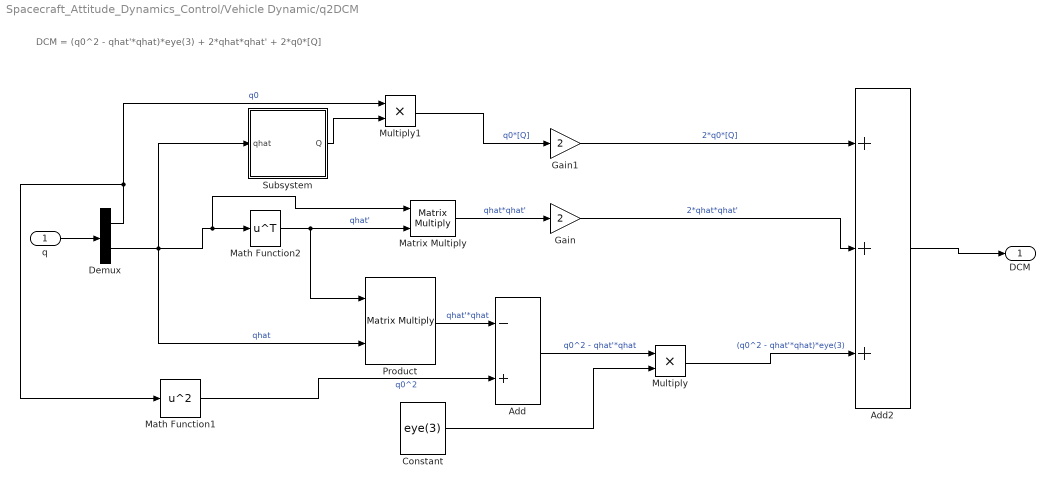
== system Spacecraft_Attitude_Dynamics_Control/Vehicle Dynamic/q2DCM ==
  note: DCM = (q0^2 - qhat'*qhat)*eye(3) + 2*qhat*qhat' + 2*q0*[Q]
  q : Inport  PortDimensions=[4,1]
  Add : Sum  Inputs=-+
  Add2 : Sum  Inputs=+++
  Constant : Constant  Value=eye(3)
  Demux : Demux  Outputs=[1,3]
  Gain : Gain  Gain=2
  Gain1 : Gain  Gain=2
  Math Function1 : Math  Operator=square  SignedPower=on  SaturateOnIntegerOverflow=on
  Math Function2 : Math  Operator=transpose  SignedPower=on  SaturateOnIntegerOverflow=on
  Matrix Multiply : Product  Multiplication=Matrix(*)
  Multiply : Product
  Multiply1 : Product
  Product : Product  Multiplication=Matrix(*)
  Subsystem : Subsystem
  DCM : Outport  VectorParamsAs1DForOutWhenUnconnected=off
  wires:
  q/1 -> Demux/1
  Demux/1 -> Math Function1/1, Multiply1/1  "q0"
  Product/1 -> Add/1  "qhat'*qhat"
  Math Function1/1 -> Add/2  "q0^2"
  Matrix Multiply/1 -> Gain/1  "qhat*qhat'"
  Subsystem/1(Q) -> Multiply1/2
  Add/1 -> Multiply/1  "q0^2 - qhat'*qhat"
  Gain/1 -> Add2/2  "2*qhat*qhat'"
  Multiply1/1 -> Gain1/1  "q0*[Q]"
  Gain1/1 -> Add2/1  "2*q0*[Q]"
  Add2/1 -> DCM/1
  Constant/1 -> Multiply/2
  Multiply/1 -> Add2/3  "(q0^2 - qhat'*qhat)*eye(3)"
  Demux/2 -> Matrix Multiply/1, Math Function2/1, Subsystem/1(qhat), Product/2  "qhat"
  Math Function2/1 -> Product/1, Matrix Multiply/2  "qhat'"

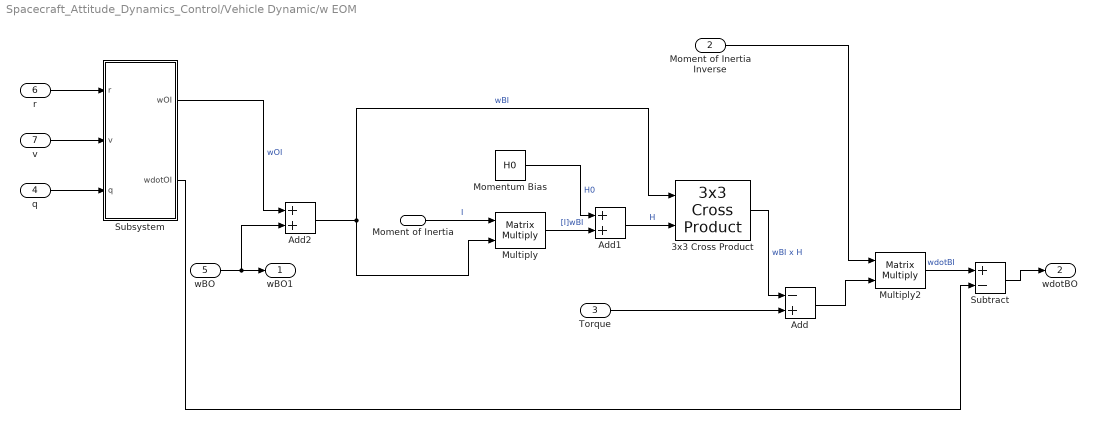
== system Spacecraft_Attitude_Dynamics_Control/Vehicle Dynamic/w EOM ==
  Moment of Inertia : Inport
  Moment of Inertia Inverse : Inport  Port=2
  Torque : Inport  Port=3
  q : Inport  Port=4
  "wBO " : Inport  Port=5
  r : Inport  Port=6
  "v " : Inport  Port=7
  3x3 Cross Product : sharedutil/3x3 Cross Product  aMode=aMode
      settings: SourceProductBaseCode=AE,PW,MT,VE,VP
  Add : Sum  Inputs=-+
  Add1 : Sum
  Add2 : Sum
  Momentum Bias : Constant  Value=H0
  Multiply : Product  Multiplication=Matrix(*)
  Multiply2 : Product  Multiplication=Matrix(*)
  Subsystem : Subsystem
  Subtract : Sum  Inputs=+-
  wBO1 : Outport  VectorParamsAs1DForOutWhenUnconnected=off
  wdotBO : Outport  Port=2  VectorParamsAs1DForOutWhenUnconnected=off
  wires:
  Moment of Inertia/1 -> Multiply/1  "I"
  Add2/1 -> 3x3 Cross Product/1, Multiply/2  "wBI"
  Torque/1 -> Add/2
  3x3 Cross Product/1 -> Add/1  "wBI x H"
  Add/1 -> Multiply2/2
  Moment of Inertia Inverse/1 -> Multiply2/1
  Multiply2/1 -> Subtract/1  "wdotBI"
  Multiply/1 -> Add1/2  "[I]wBI"
  Momentum Bias/1 -> Add1/1  "H0"
  Add1/1 -> 3x3 Cross Product/2  "H"
  r/1 -> Subsystem/1(r)
  "v "/1 -> Subsystem/2(v)
  Subsystem/1(wOI) -> Add2/1  "wOI"
  q/1 -> Subsystem/3(q)
  "wBO "/1 -> wBO1/1, Add2/2
  Subsystem/2(wdotOI) -> Subtract/2
  Subtract/1 -> wdotBO/1

== system Spacecraft_Attitude_Dynamics_Control/Animation/Earth Rotation/q2eulerparameters ==
  q : Inport
  Demux : Demux  Outputs=[1,3]
  Divide : Product  Inputs=/*
  Gain : Gain  Gain=2
  Mux : Mux  Inputs=2
  Trigonometric Function : Trigonometry  Operator=acos
  Trigonometric Function1 : Trigonometry
  e,phi : Outport  VectorParamsAs1DForOutWhenUnconnected=off
  wires:
  Demux/2 -> Divide/2  "qhat"
  Trigonometric Function1/1 -> Divide/1
  Divide/1 -> Mux/1  "e"
  Trigonometric Function/1 -> Trigonometric Function1/1, Gain/1  "phi/2"
  Demux/1 -> Trigonometric Function/1  "q0"
  Gain/1 -> Mux/2  "phi"
  Mux/1 -> e,phi/1
  q/1 -> Demux/1

== system Spacecraft_Attitude_Dynamics_Control/Vehicle Dynamic/q propagation/If Action Subsystem ==
  ||beta||/2 : Inport
  Action Port : ActionPort  ActionPortLabel=else
  Divide : Product  Inputs=*/
  Trigonometric Function : Trigonometry
  (2/||beta||)*sin(||beta||/2) : Outport  VectorParamsAs1DForOutWhenUnconnected=off
  wires:
  ||beta||/2/1 -> Trigonometric Function/1, Divide/2
  Trigonometric Function/1 -> Divide/1
  Divide/1 -> (2/||beta||)*sin(||beta||/2)/1

== system Spacecraft_Attitude_Dynamics_Control/Vehicle Dynamic/q propagation/If Action Subsystem1 ==
  Action Port : ActionPort  ActionPortLabel=if(u1 < 1e-10)
  Constant : Constant  Value=0
  Zero : Outport  InitialOutput=0  VectorParamsAs1DForOutWhenUnconnected=off
  wires:
  Constant/1 -> Zero/1

== system Spacecraft_Attitude_Dynamics_Control/Vehicle Dynamic/q2DCM/Subsystem ==
  qhat : Inport
  Bus Creator : BusCreator  Inputs=7
  Bus Selector : BusSelector  OutputSignals=0,-q3,q2  OutputAsBus=on
  Bus Selector1 : BusSelector  OutputSignals=q3,0,-q1  OutputAsBus=on
  Bus Selector2 : BusSelector  OutputSignals=-q2,q1,0  OutputAsBus=on
  Constant : Constant  Value=0
  Demux1 : Demux  Outputs=3
  Demux2 : Demux  Outputs=3
  Display : Display
  Gain : Gain  Gain=-1
  Vector Concatenate : Concatenate  NumInputs=3  Mode=Multidimensional array  ConcatenateDimension=2
  Q : Outport  VectorParamsAs1DForOutWhenUnconnected=off
  wires:
  Demux1/3 -> Bus Creator/4  "q3"
  Bus Creator/1 -> Bus Selector2/1, Bus Selector1/1, Bus Selector/1
  Demux2/1 -> Bus Creator/5  "-q1"
  Bus Selector2/1 -> Vector Concatenate/3
  qhat/1 -> Gain/1, Demux1/1
  Demux1/2 -> Bus Creator/3  "q2"
  Demux2/3 -> Bus Creator/7  "-q3"
  Bus Selector1/1 -> Vector Concatenate/2
  Demux2/2 -> Bus Creator/6  "-q2"
  Demux1/1 -> Bus Creator/2  "q1"
  Gain/1 -> Demux2/1
  Bus Selector/1 -> Vector Concatenate/1
  Constant/1 -> Bus Creator/1  "0"
  Vector Concatenate/1 -> Display/1, Q/1

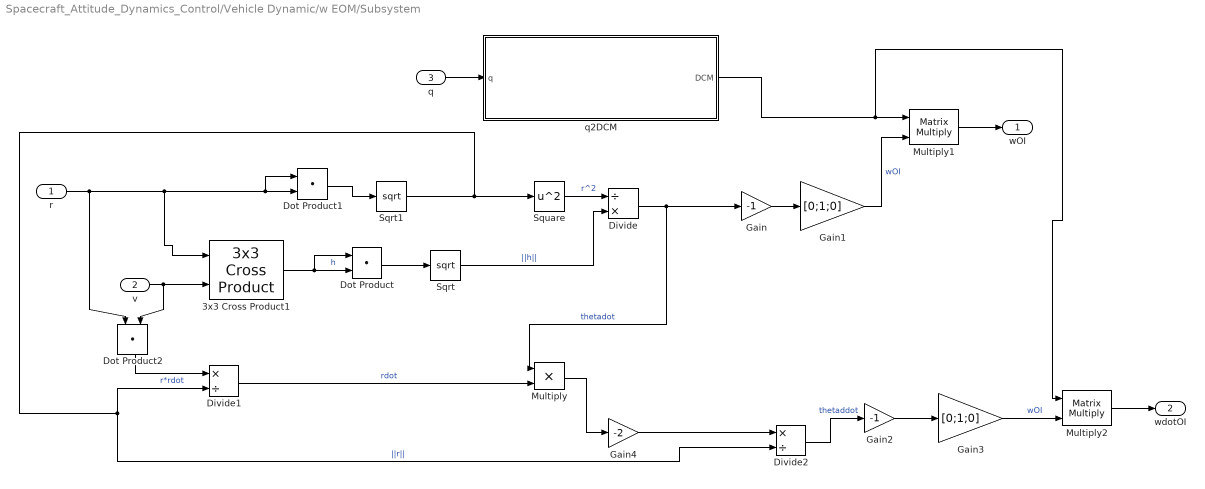
== system Spacecraft_Attitude_Dynamics_Control/Vehicle Dynamic/w EOM/Subsystem ==
  r : Inport
  v : Inport  Port=2
  q : Inport  Port=3
  3x3 Cross Product1 : sharedutil/3x3 Cross Product  aMode=aMode
      settings: SourceProductBaseCode=AE,PW,MT,VE,VP
  Divide : Product  Inputs=/*
  Divide1 : Product  Inputs=*/
  Divide2 : Product  Inputs=*/
  Dot Product : DotProduct  InputSameDT=on  OutDataTypeStr=Inherit: Inherit via internal rule
  Dot Product1 : DotProduct  InputSameDT=on  OutDataTypeStr=Inherit: Inherit via internal rule
  Dot Product2 : DotProduct  InputSameDT=on  OutDataTypeStr=Inherit: Inherit via internal rule
  Gain : Gain  Gain=-1
  Gain1 : Gain  Gain=[0;1;0]
  Gain2 : Gain  Gain=-1
  Gain3 : Gain  Gain=[0;1;0]
  Gain4 : Gain  Gain=-2
  Multiply : Product
  Multiply1 : Product  Multiplication=Matrix(*)
  Multiply2 : Product  Multiplication=Matrix(*)
  Sqrt : Sqrt  SaturateOnIntegerOverflow=on
  Sqrt1 : Sqrt  SaturateOnIntegerOverflow=on
  Square : Math  Operator=square  SignedPower=on  SaturateOnIntegerOverflow=on
  q2DCM : Subsystem
  wOI : Outport  VectorParamsAs1DForOutWhenUnconnected=off
  wdotOI : Outport  Port=2  VectorParamsAs1DForOutWhenUnconnected=off
  wires:
  r/1 -> Dot Product2/1, 3x3 Cross Product1/1, Dot Product1/1, Dot Product1/2
  Sqrt/1 -> Divide/2  "||h||"
  Dot Product/1 -> Sqrt/1
  Divide/1 -> Multiply/1, Gain/1  "thetadot"
  Sqrt1/1 -> Divide2/2, Divide1/2, Square/1  "||r||"
  3x3 Cross Product1/1 -> Dot Product/1, Dot Product/2  "h"
  Square/1 -> Divide/1  "r^2"
  Gain/1 -> Gain1/1
  Dot Product1/1 -> Sqrt1/1
  v/1 -> 3x3 Cross Product1/2, Dot Product2/2
  q2DCM/1(DCM) -> Multiply2/1, Multiply1/1
  q/1 -> q2DCM/1(q)
  Gain1/1 -> Multiply1/2  "wOI"
  Multiply1/1 -> wOI/1
  Gain2/1 -> Gain3/1
  Gain3/1 -> Multiply2/2  "wOI"
  Multiply2/1 -> wdotOI/1
  Dot Product2/1 -> Divide1/1  "r*rdot"
  Divide1/1 -> Multiply/2  "rdot"
  Multiply/1 -> Gain4/1
  Gain4/1 -> Divide2/1
  Divide2/1 -> Gain2/1  "thetaddot"

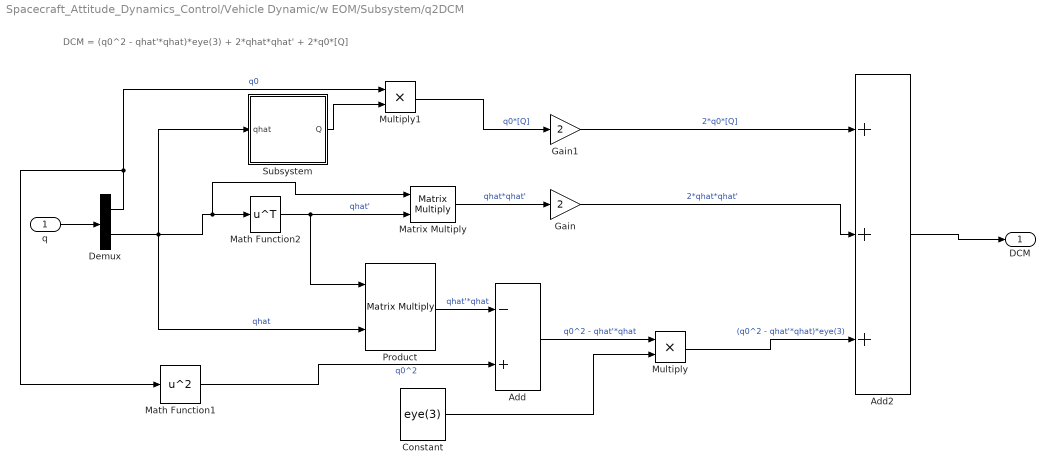
== system Spacecraft_Attitude_Dynamics_Control/Vehicle Dynamic/w EOM/Subsystem/q2DCM ==
  note: DCM = (q0^2 - qhat'*qhat)*eye(3) + 2*qhat*qhat' + 2*q0*[Q]
  q : Inport  PortDimensions=[4,1]
  Add : Sum  Inputs=-+
  Add2 : Sum  Inputs=+++
  Constant : Constant  Value=eye(3)
  Demux : Demux  Outputs=[1,3]
  Gain : Gain  Gain=2
  Gain1 : Gain  Gain=2
  Math Function1 : Math  Operator=square  SignedPower=on  SaturateOnIntegerOverflow=on
  Math Function2 : Math  Operator=transpose  SignedPower=on  SaturateOnIntegerOverflow=on
  Matrix Multiply : Product  Multiplication=Matrix(*)
  Multiply : Product
  Multiply1 : Product
  Product : Product  Multiplication=Matrix(*)
  Subsystem : Subsystem
  DCM : Outport  VectorParamsAs1DForOutWhenUnconnected=off
  wires:
  q/1 -> Demux/1
  Demux/1 -> Math Function1/1, Multiply1/1  "q0"
  Product/1 -> Add/1  "qhat'*qhat"
  Math Function1/1 -> Add/2  "q0^2"
  Matrix Multiply/1 -> Gain/1  "qhat*qhat'"
  Subsystem/1(Q) -> Multiply1/2
  Add/1 -> Multiply/1  "q0^2 - qhat'*qhat"
  Gain/1 -> Add2/2  "2*qhat*qhat'"
  Multiply1/1 -> Gain1/1  "q0*[Q]"
  Gain1/1 -> Add2/1  "2*q0*[Q]"
  Add2/1 -> DCM/1
  Constant/1 -> Multiply/2
  Multiply/1 -> Add2/3  "(q0^2 - qhat'*qhat)*eye(3)"
  Demux/2 -> Matrix Multiply/1, Math Function2/1, Subsystem/1(qhat), Product/2  "qhat"
  Math Function2/1 -> Product/1, Matrix Multiply/2  "qhat'"

== system Spacecraft_Attitude_Dynamics_Control/Vehicle Dynamic/w EOM/Subsystem/q2DCM/Subsystem ==
  qhat : Inport
  Bus Creator : BusCreator  Inputs=7
  Bus Selector : BusSelector  OutputSignals=0,-q3,q2  OutputAsBus=on
  Bus Selector1 : BusSelector  OutputSignals=q3,0,-q1  OutputAsBus=on
  Bus Selector2 : BusSelector  OutputSignals=-q2,q1,0  OutputAsBus=on
  Constant : Constant  Value=0
  Demux1 : Demux  Outputs=3
  Demux2 : Demux  Outputs=3
  Display : Display
  Gain : Gain  Gain=-1
  Vector Concatenate : Concatenate  NumInputs=3  Mode=Multidimensional array  ConcatenateDimension=2
  Q : Outport  VectorParamsAs1DForOutWhenUnconnected=off
  wires:
  Demux1/3 -> Bus Creator/4  "q3"
  Bus Creator/1 -> Bus Selector2/1, Bus Selector1/1, Bus Selector/1
  Demux2/1 -> Bus Creator/5  "-q1"
  Bus Selector2/1 -> Vector Concatenate/3
  qhat/1 -> Gain/1, Demux1/1
  Demux1/2 -> Bus Creator/3  "q2"
  Demux2/3 -> Bus Creator/7  "-q3"
  Bus Selector1/1 -> Vector Concatenate/2
  Demux2/2 -> Bus Creator/6  "-q2"
  Demux1/1 -> Bus Creator/2  "q1"
  Gain/1 -> Demux2/1
  Bus Selector/1 -> Vector Concatenate/1
  Constant/1 -> Bus Creator/1  "0"
  Vector Concatenate/1 -> Display/1, Q/1
